simulink model "untitled"  (Simulink 7.9)
settings: Solver=FixedStepDiscrete  SolverMode=SingleTasking  StartTime=0.0  StopTime=1/48000  RelTol=1e-3
undefined symbols (not defined in the file or in its folder): D, dfilt, Fs, get, j, sided, Two
libraries: dspobslib x3, dsparch4 x1, commrandsrc2 x1, dspxfrm3 x1, dspsigops x1, dspstat3 x1, dspsnks4 x1
settings Model: Creator=Estilo  LastModifiedBy=Estilo

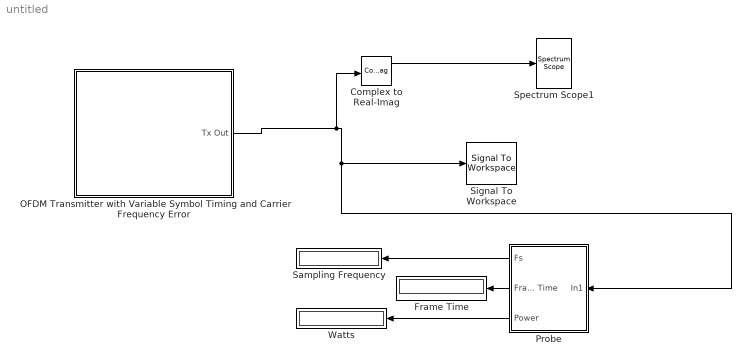
== system untitled ==
  Complex to Real-Imag : ComplexToRealImag
  Frame Time : Display
  OFDM Transmitter with Variable Symbol Timing and Carrier Frequency Error : Subsystem
  Probe : Subsystem
  Sampling Frequency : Display
  Signal To Workspace : SignalToWorkspace  VariableName=yout1
      settings: CopyFcn=dspblkcopystw(gcbh);
  Spectrum Scope1 : dspsnks4/Spectrum Scope  ScopeProperties=on  Domain=Frequency  HorizSpan=1  UseBuffer=on  BufferSize=160  Overlap=0  TreatMby1Signals=One channel  inpFftLenInherit=on  FFTlength=512  numAvg=1  DisplayProperties=off  AxisGrid=on  Memory=off  FrameNumber=on  AxisLegend=off  AxisZoom=off  OpenScopeAtSimStart=on  OpenScopeImmediately=off  FigPos=get(0,'defaultfigureposition')  AxisProperties=off  XUnits=Hertz  XRange=Two-sided ((-Fs/2...Fs/2])  XDisplay=0  InheritXIncr=on  XIncr=1.0  XLabel=Samples  XLimit=User-defined  YUnits=dBW/Hertz  XMax=24000  XMin=-24000  YLabel=Magnitude-squared, dB  LineProperties=off  wintypeSpecScope=Boxcar  RsSpecScope=50  betaSpecScope=5  winsampSpecScope=Periodic  XAxisParamsVer=6.9  isFrameUpgraded=on
      settings: YMin=-93.1497  YMax=-21.8265
  Watts : Display
  wires:
  OFDM Transmitter with Variable Symbol Timing and Carrier Frequency Error/1(Tx Out) -> Complex to Real-Imag/1, Probe/1(In1), Signal To Workspace/1
  Complex to Real-Imag/1 -> Spectrum Scope1/1
  Probe/2(Frame Time) -> Frame Time/1
  Probe/1(Fs) -> Sampling Frequency/1
  Probe/3(Power) -> Watts/1

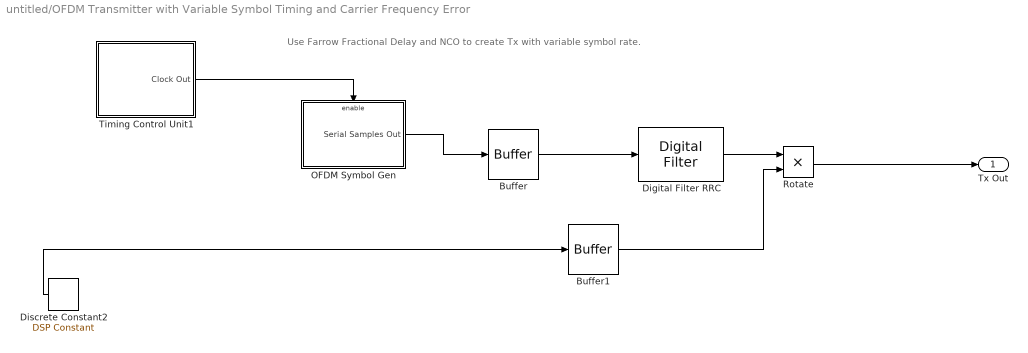
== system untitled/OFDM Transmitter with Variable Symbol Timing and Carrier Frequency Error ==
  note: Use Farrow Fractional Delay and NCO to create Tx with variable symbol rate.
  Buffer : Buffer  N=160
  Buffer1 : Buffer  N=160
  "Digital Filter RRC " : dsparch4/Digital Filter  TypePopup=FIR (all zeros)  IIRFiltStruct=Direct form II transposed  AllPoleFiltStruct=Direct form  FIRFiltStruct=Direct form  CoeffSource=Specify via dialog  NumCoeffs=Cofff  DenCoeffs=[1 0.1]  BiQuadCoeffs=[1 0.3 0.4 1 0.1 0.2]  LatticeCoeffs=[0.2 0.4]  denIgnore=on  FiltPerSampPopup=One filter per frame  IC=0  ICnum=0  ICden=0  roundingMode=Floor  overflowMode=off  ScaleValues=1  scaleValueFracLength=14  stageInFracLength=15  stageOutFracLength=15  FilterSource=Specify via dialog  dfiltObjectName=dfilt.dffir([1 2 1])  InputProcessing=Inherited (this choice will be removed - see release notes)
  Discrete Constant2 : dspobslib/DSP Constant  Value=1  SampleMode=Discrete  discreteOutput=Sample-based (interpret vectors as 1-D)  continuousOutput=Sample-based  sampTime=1/48000  framePeriod=inf  dataType=Inherit via back propagation  isSigned=on  wordLen=16  udDataType=sfix(16)  fracBitsMode=Best precision  numFracBits=15  InterpretAs1D=on  Ts=inf  FramebasedOutput=off
      settings: additionalParams=on
  OFDM Symbol Gen : Subsystem
  Rotate : Product  RndMeth=Zero
  Timing Control Unit1 : Subsystem
  Tx Out : Outport
  wires:
  Discrete Constant2/1 -> Buffer1/1
  Rotate/1 -> Tx Out/1
  OFDM Symbol Gen/1(Serial Samples Out) -> Buffer/1
  Timing Control Unit1/1(Clock Out) -> OFDM Symbol Gen/Enable
  "Digital Filter RRC "/1 -> Rotate/1
  Buffer1/1 -> Rotate/2
  Buffer/1 -> "Digital Filter RRC "/1

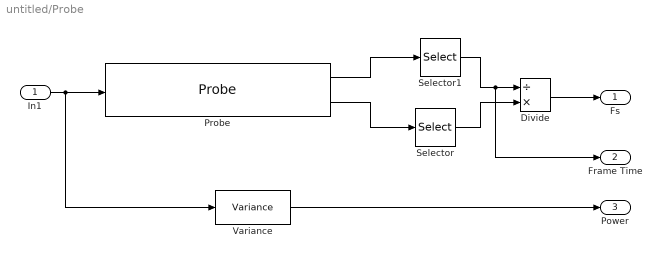
== system untitled/Probe ==
  In1 : Inport
  Divide : Product  Inputs=/*
  Probe : Probe  ProbeWidth=off  ProbeComplexSignal=off  ProbeSignalDimensions=on
  Selector : Selector  InputPortWidth=2  IndexOptions=Index vector (dialog)  Indices=[1]  OutputSizes=1
  Selector1 : Selector  InputPortWidth=2  IndexOptions=Index vector (dialog)  Indices=[1]  OutputSizes=1
  Variance : dspstat3/Variance  run=off  reset_popup=None  InputProcessing=Columns as channels (frame based)  directionMode=Each column  dimension=1  treatSBRowAsCol=on  roiEnable=off  roiType=Rectangles  roiPortion=Entire ROI  roiOutput=Individual statistics for each ROI  roiFlag=off  roundingMode=Floor  overflowMode=off
  Fs : Outport
  Frame Time : Outport  Port=2
  Power : Outport  Port=3
  wires:
  In1/1 -> Probe/1, Variance/1
  Divide/1 -> Fs/1
  Selector/1 -> Divide/2
  Selector1/1 -> Divide/1, Frame Time/1
  Probe/1 -> Selector1/1
  Probe/2 -> Selector/1
  Variance/1 -> Power/1

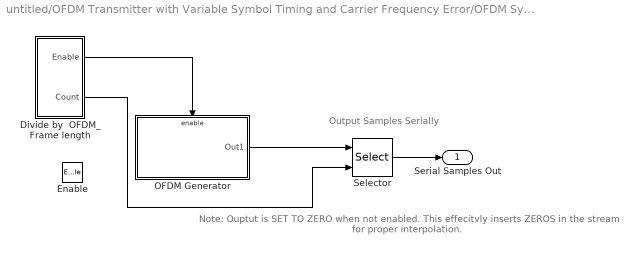
== system untitled/OFDM Transmitter with Variable Symbol Timing and Carrier Frequency Error/OFDM Symbol Gen ==
  note: Note: Ouptut is SET TO ZERO
      | when not enabled.
      | This effecitvly inserts ZEROS in the stream
      | for proper interpolation.
  note: Output Samples Serially
  Enable : EnablePort
  Divide by  OFDM_Frame length : Subsystem  TreatAsAtomicUnit=on  mask(Pulse Divider){div=160, ph=0}
      mask prompts: div "Modulo:"; ph "Initial Phase Delay (cycles):"
  OFDM Generator : Subsystem
  Selector : Selector  InputPortWidth=160  IndexOptions=Index vector (port)  Indices=[1 3]  OutputSizes=1
  Serial Samples Out : Outport  OutputWhenDisabled=reset  InitialOutput=0+j*eps
  wires:
  Divide by  OFDM_Frame length/2(Count) -> Selector/2
  Selector/1 -> Serial Samples Out/1
  Divide by  OFDM_Frame length/1(Enable) -> OFDM Generator/Enable
  OFDM Generator/1(Out1) -> Selector/1

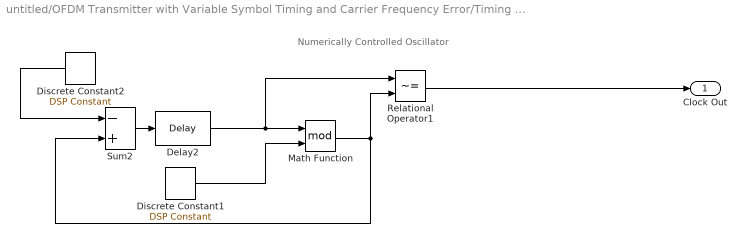
== system untitled/OFDM Transmitter with Variable Symbol Timing and Carrier Frequency Error/Timing Control Unit1 ==
  note: Numerically Controlled Oscillator
  Delay2 : dspsigops/Delay  InputProcessing=Inherited (this choice will be removed - see release notes)  dly_unit=Samples  delay=1  ic_detail=on  dif_ic_for_ch=off  dif_ic_for_dly=off  ic=0  reset_popup=None
  Discrete Constant1 : dspobslib/DSP Constant  Value=1  SampleMode=Discrete  discreteOutput=Sample-based (interpret vectors as 1-D)  continuousOutput=Sample-based  sampTime=inf  framePeriod=inf  dataType=Inherit via back propagation  isSigned=on  wordLen=16  udDataType=sfix(16)  fracBitsMode=Best precision  numFracBits=15  InterpretAs1D=on  Ts=inf  FramebasedOutput=off
      settings: additionalParams=on
  Discrete Constant2 : dspobslib/DSP Constant  Value=1/D  SampleMode=Discrete  discreteOutput=Sample-based (interpret vectors as 1-D)  continuousOutput=Sample-based  sampTime=inf  framePeriod=inf  dataType=Inherit via back propagation  isSigned=on  wordLen=16  udDataType=sfix(16)  fracBitsMode=Best precision  numFracBits=15  InterpretAs1D=on  Ts=inf  FramebasedOutput=off
      settings: additionalParams=on
  Math Function : Math  Operator=mod  SaturateOnIntegerOverflow=on
  Relational Operator1 : RelationalOperator  Operator=~=  OutDataTypeStr=boolean
  Sum2 : Sum  Inputs=-+  SaturateOnIntegerOverflow=on  InputSameDT=on  OutDataTypeStr=Inherit: Same as first input
  Clock Out : Outport
  wires:
  Discrete Constant2/1 -> Sum2/1
  Relational Operator1/1 -> Clock Out/1
  Math Function/1 -> Sum2/2, Relational Operator1/2
  Sum2/1 -> Delay2/1
  Discrete Constant1/1 -> Math Function/2
  Delay2/1 -> Relational Operator1/1, Math Function/1

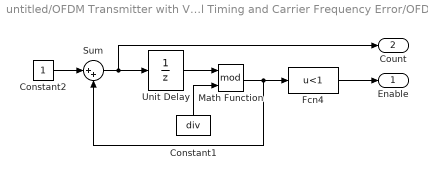
== system untitled/OFDM Transmitter with Variable Symbol Timing and Carrier Frequency Error/OFDM Symbol Gen/Divide by  OFDM_Frame length ==
  Constant1 : Constant  Value=div
  Constant2 : Constant
  Fcn4 : Fcn  Expr=u<1
  Math Function : Math  Operator=mod  SaturateOnIntegerOverflow=on
  Sum : Sum  Inputs=|++  SaturateOnIntegerOverflow=on  InputSameDT=on  OutDataTypeStr=Inherit: Same as first input
  Unit Delay : UnitDelay  X0=div-ph  SampleTime=-1
  Enable : Outport
  Count : Outport  Port=2
  wires:
  Fcn4/1 -> Enable/1
  Constant1/1 -> Math Function/2
  Math Function/1 -> Fcn4/1, Sum/2
  Unit Delay/1 -> Math Function/1
  Constant2/1 -> Sum/1
  Sum/1 -> Count/1, Unit Delay/1

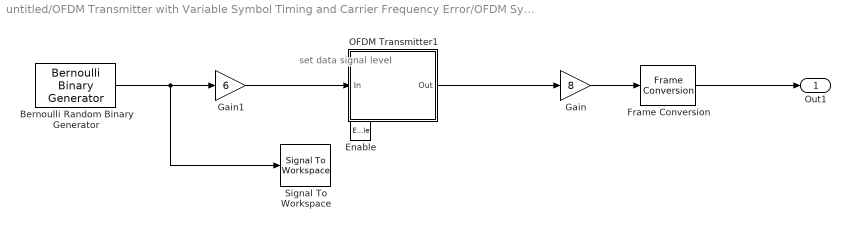
== system untitled/OFDM Transmitter with Variable Symbol Timing and Carrier Frequency Error/OFDM Symbol Gen/OFDM Generator ==
  note: set data signal level
  Enable : EnablePort
  Bernoulli Random Binary Generator : commrandsrc2/Bernoulli Binary Generator  P=0.5  seed=123  Ts=1/1000  frameBased=on  sampPerFrame=4  orient=off  outDataType=double
  Frame Conversion : FrameConversion  OutFrame=Sample-based
  Gain : Gain  Gain=8
  Gain1 : Gain  Gain=6  SaturateOnIntegerOverflow=on  OutDataTypeStr=Inherit: Same as input  ParamDataTypeStr=Inherit: Same as input
  OFDM Transmitter1 : Subsystem
      mask Display: disp('OFDM\nTransmitter')
  Signal To Workspace : SignalToWorkspace  VariableName=yout3
      settings: CopyFcn=dspblkcopystw(gcbh);
  Out1 : Outport
  wires:
  Gain1/1 -> OFDM Transmitter1/1(In)
  Gain/1 -> Frame Conversion/1
  OFDM Transmitter1/1(Out) -> Gain/1
  Bernoulli Random Binary Generator/1 -> Gain1/1, Signal To Workspace/1
  Frame Conversion/1 -> Out1/1

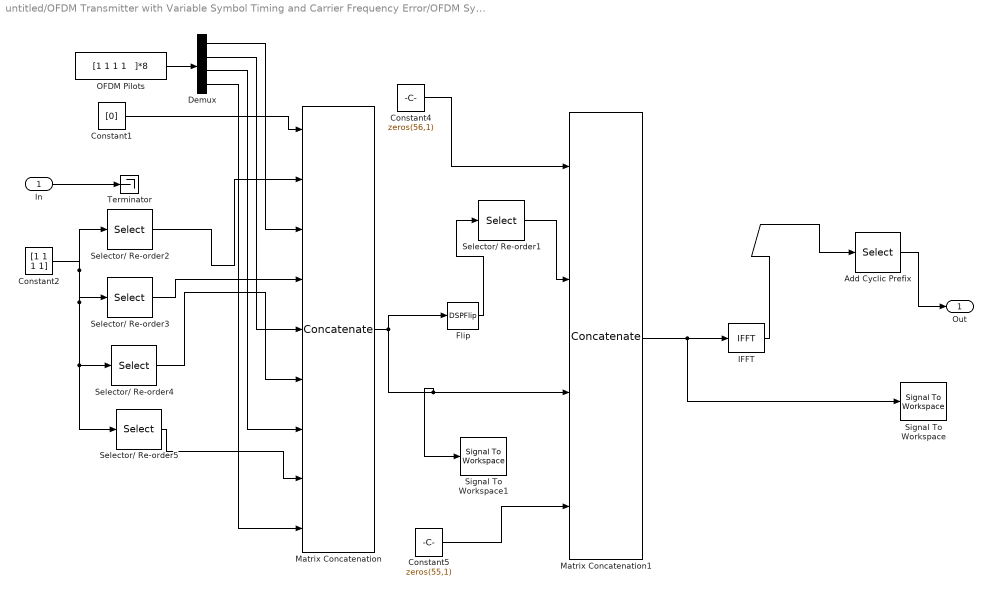
== system untitled/OFDM Transmitter with Variable Symbol Timing and Carrier Frequency Error/OFDM Symbol Gen/OFDM Generator/OFDM Transmitter1 ==
  In : Inport
  Add Cyclic Prefix : Selector  InputPortWidth=128  IndexOptions=Index vector (dialog)  Indices=[97:128 1:128]  OutputSizes=1
  Constant1 : Constant  Value=[0]
  Constant2 : Constant  Value=[1 1 1 1]
  Constant4 : Constant  Value=zeros(56,1)
  Constant5 : Constant  Value=zeros(55,1)
  Demux : Demux
  Flip : DSPFlip
  IFFT : dspxfrm3/IFFT  CompMethod=Table lookup  TableOpt=HYBRID  TableOptActive=Speed  BitRevOrder=off  cs_in=off  SkipNorm=on  InheritFFTLength=on  FFTLength=64  mode=Complex  outSamplingMode=Frame based  RowConvenienceOn=on  FFTImplementation=Auto  firstCoeffDataTypeStr=Inherit: Same word length as input  firstCoeffLastDataTypeStr=Inherit: Same word length as input  outputMin=[]  outputMax=[]  roundingMode=Floor  overflowMode=off
  Matrix Concatenation : Concatenate  NumInputs=9  Mode=Multidimensional array
  Matrix Concatenation1 : Concatenate  NumInputs=4  Mode=Multidimensional array
  OFDM Pilots : Constant  Value="[1 1 1 1   ]*8"
  Selector/ Re-order1 : Selector  InputPortWidth=9  IndexOptions=Index vector (dialog)  Indices=[1:8]  OutputSizes=1
  Selector/ Re-order2 : Selector  InputPortWidth=4  IndexOptions=Index vector (dialog)  Indices=[1]  OutputSizes=1
  Selector/ Re-order3 : Selector  InputPortWidth=4  IndexOptions=Index vector (dialog)  Indices=[2]  OutputSizes=1
  Selector/ Re-order4 : Selector  InputPortWidth=4  IndexOptions=Index vector (dialog)  Indices=[3]  OutputSizes=1
  Selector/ Re-order5 : Selector  InputPortWidth=4  IndexOptions=Index vector (dialog)  Indices=[4]  OutputSizes=1
  Signal To Workspace : SignalToWorkspace  VariableName=yout2
      settings: CopyFcn=dspblkcopystw(gcbh);
  Signal To Workspace1 : SignalToWorkspace  VariableName=yout
      settings: CopyFcn=dspblkcopystw(gcbh);
  Terminator : Terminator
  Out : Outport
  wires:
  Add Cyclic Prefix/1 -> Out/1
  Matrix Concatenation1/1 -> IFFT/1, Signal To Workspace/1
  Constant5/1 -> Matrix Concatenation1/4
  Selector/ Re-order1/1 -> Matrix Concatenation1/2
  Flip/1 -> Selector/ Re-order1/1
  Matrix Concatenation/1 -> Signal To Workspace1/1, Matrix Concatenation1/3, Flip/1
  Constant4/1 -> Matrix Concatenation1/1
  Demux/4 -> Matrix Concatenation/9
  Demux/3 -> Matrix Concatenation/7
  Demux/2 -> Matrix Concatenation/5
  Demux/1 -> Matrix Concatenation/3
  OFDM Pilots/1 -> Demux/1
  Selector/ Re-order2/1 -> Matrix Concatenation/2
  Constant1/1 -> Matrix Concatenation/1
  IFFT/1 -> Add Cyclic Prefix/1
  Selector/ Re-order3/1 -> Matrix Concatenation/4
  Selector/ Re-order4/1 -> Matrix Concatenation/6
  Selector/ Re-order5/1 -> Matrix Concatenation/8
  In/1 -> Terminator/1
  Constant2/1 -> Selector/ Re-order5/1, Selector/ Re-order4/1, Selector/ Re-order3/1, Selector/ Re-order2/1
